simulink model "Copy_of_read_ADC_scribe_PWM_ROB_1ver"  (R2024a)
settings: Solver=ode8  StartTime=0.0  StopTime=400  FixedStep=Ts  RelTol=1e-3  EnableMultiTasking=on
values from neighbouring files (symbols this model uses):
  am = 200    [parameters.m]
  bm = 1    [parameters.m]
  C = 790*10^(-6)    (= 0.00079)    [parameters.m]
  k1 = 8000    [parameters.m]
  k2 = 15    [parameters.m]
  kapam = 1    [parameters.m]
  L = 2000*10^(-6)    (= 0.002)    [parameters.m]
  Qaster = bm    (= 1)    [parameters.m]
  R = 10000    [parameters.m]
  Ts = 0.01    [parameters.m]
  x2d_dot = 0    [parameters.m]
undefined symbols (not defined in the file or in its folder): Down, GPTRIP1SEL, GPTRIP2SEL, TZ1, TZ2, Up
libraries: c2802xlib x5
settings Model: SimulationMode=external  ExtModeTrigDuration=8  Creator=omar_  LastModifiedBy=rodol
settings DataIOCC: LimitDataPoints=on  MaxDataPoints=1000000  SaveFormat=StructureWithTime  InspectSignalLogs=on
settings OptimizationCC: DefaultUnderspecifiedDataType=single  EnhancedBackFolding=on  PassReuseOutputArgsAs=Individual arguments  MaxStackSize=1024  OptimizeBlockOrder=speed  DifferentSizesBufferReuse=on  OptimizationCustomize=off  DenormalBehavior=FlushToZero  EfficientTunableParamExpr=on
settings DebuggingCC: ParameterTunabilityLossMsg=error  UnconnectedInputMsg=warning  UnconnectedOutputMsg=warning  UnconnectedLineMsg=warning
settings HardwareCC: ProdBitPerChar=16  ProdBitPerInt=16  ProdBitPerPointer=32  ProdBitPerSizeT=32  ProdBitPerPtrDiffT=32  ProdLargestAtomicInteger=Integer  ProdLargestAtomicFloat=None  ProdWordSize=16  ProdLongLongMode=on  ProdHWDeviceType=Texas Instruments->C2000
settings ModelReferenceCC: EnableRefExpFcnMdlSchedulingChecks=on
settings SFSimCC: MATLABDynamicMemAlloc=off
settings RTWCC: Description=Embedded Coder  SystemTargetFile=ert.tlc  HardwareBoard=TI Delfino F28379D LaunchPad  TemplateMakefile=ert_default_tmf  Toolchain=Texas Instruments Code Composer Studio (C2000)  GPUComputeCapability=3.5  DLArmComputeVersion=19.05
settings CodeAppCC: ForceParamTrailComments=on  IgnoreCustomStorageClasses=off  OperatorAnnotations=on  SimulinkDataObjDesc=on  SFDataObjDesc=on  InsertBlockDesc=on
settings ERTTargetCC: CodeReplacementLibrary=TI C28x  SupportContinuousTime=on  ExtMode=on  ExtModeTransport=3  ExtModeStaticAllocSize=10000  ExtModeMexArgs='127.0.0.1' 0 17725

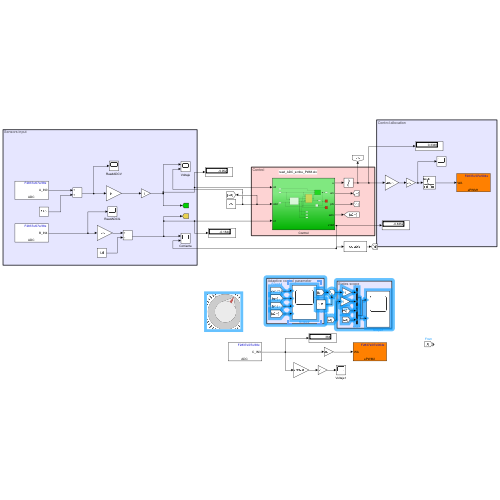
[thumbnail: Simulink's stored preview of the top-level diagram]
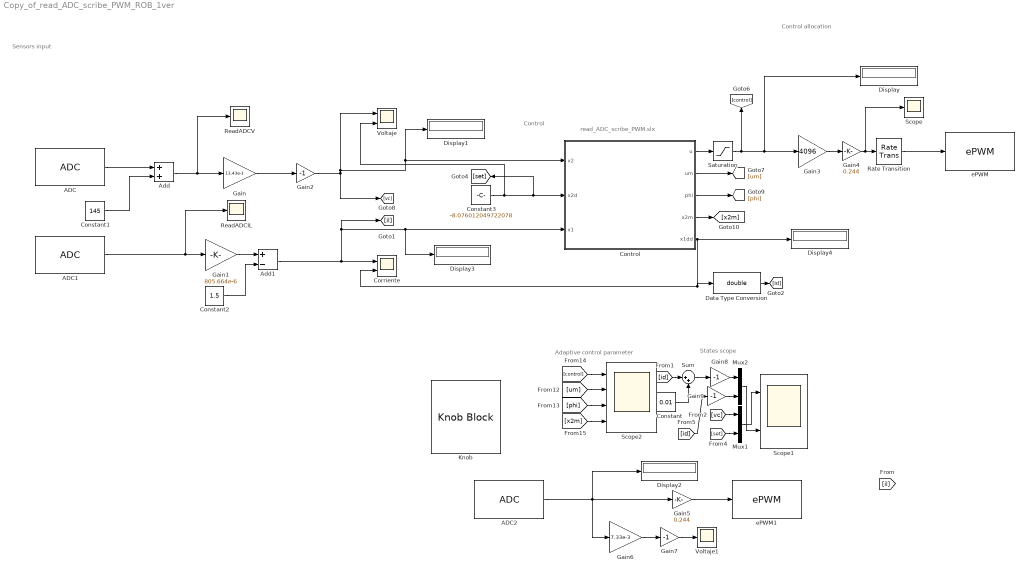
== system Copy_of_read_ADC_scribe_PWM_ROB_1ver ==
  note: Sensors input
  note: Control allocation
  note: read_ADC_scribe_PWM.slx
  note: Control
  note: Adaptive control parameter
  note: States scope
  ADC : c2802xlib/ADC  blkParamProc=C2000_Type4  ADCModule=A  samplingMode=Single sample mode  ADCResolution=12-bit (Single-ended input)  useSOC1=SOC0  useSOC2=SOC0_SOC1  SOCAcquisitionWindow=15  SOCTriggerSource=Software  SOCInterruptTrigger=No ADCINT  Ts=Ts  dType=uint16  postInterrupt=off  interruptSel=ADCINT1  ADCINTContinuous=on  endma=off  chdma=1  conv1=ADCINA0  conv2=ADCINA0 and ADCINB0  conv1_Type4=ADCIN0  conv2_Type4=ADCIN0 and ADCIN1
  ADC1 : c2802xlib/ADC  blkParamProc=C2000_Type4  ADCModule=B  samplingMode=Single sample mode  ADCResolution=12-bit (Single-ended input)  useSOC1=SOC4  useSOC2=SOC0_SOC1  SOCAcquisitionWindow=15  SOCTriggerSource=Software  SOCInterruptTrigger=No ADCINT  Ts=Ts  dType=uint16  postInterrupt=off  interruptSel=ADCINT1  ADCINTContinuous=on  endma=off  chdma=1  conv1=ADCINA0  conv2=ADCINA0 and ADCINB0  conv1_Type4=ADCIN4  conv2_Type4=ADCIN0 and ADCIN1
  ADC2 : c2802xlib/ADC  blkParamProc=C2000_Type4  ADCModule=C  samplingMode=Single sample mode  ADCResolution=12-bit (Single-ended input)  useSOC1=SOC3  useSOC2=SOC0_SOC1  SOCAcquisitionWindow=15  SOCTriggerSource=Software  SOCInterruptTrigger=No ADCINT  Ts=Ts  dType=uint16  postInterrupt=off  interruptSel=ADCINT1  ADCINTContinuous=on  endma=off  chdma=1  conv1=ADCINA0  conv2=ADCINA0 and ADCINB0  conv1_Type4=ADCIN3  conv2_Type4=ADCIN0 and ADCIN1
  Add : Sum
  Add1 : Sum  Inputs=+-
  Constant : Constant  Value=0.01
  Constant1 : Constant  Value=145
  Constant2 : Constant  Value=1.5
  Constant3 : Constant  Value=-8.076012049722078
  Control : Subsystem
  Corriente : Scope  NumInputPorts=2
  Data Type Conversion : DataTypeConversion  OutDataTypeStr=double  SaturateOnIntegerOverflow=off  RndMeth=Floor
  Display{,1..4} (5 alike) : Display
  Gain : Gain  Gain=13.43e-3  ParamDataTypeStr=double
  Gain1 : Gain  Gain=805.664e-6  ParamDataTypeStr=double
  Gain2 : Gain  Gain=-1  ParamDataTypeStr=double
  Gain3 : Gain  Gain=4096
  Gain4 : Gain  Gain=0.244
  Gain5 : Gain  Gain=0.244  OutDataTypeStr=double
  Gain6 : Gain  Gain=7.33e-3  ParamDataTypeStr=double
  Gain7 : Gain  Gain=-1  ParamDataTypeStr=double
  Gain8 : Gain  Gain=-1
  Gain9 : Gain  Gain=-1
  Knob : KnobBlock  ScaleMin=-20  ScaleMax=0
  Mux1 : Mux  Inputs=2
  Mux2 : Mux  Inputs=2
  Rate Transition : RateTransition
  ReadADCIL : Scope
  ReadADCV : Scope
  Saturation : Saturate  UpperLimit=1  LowerLimit=-50
  Scope : Scope
  Scope1 : Scope  NumInputPorts=2
  Scope2 : Scope  NumInputPorts=4
  Sum : Sum  Inputs=|++
  Voltaje : Scope  NumInputPorts=2
  Voltaje1 : Scope
  ePWM : c2802xlib/ePWM  PwmType=C2000_Type4  useModule=ePWM1  ePWMxLINKTBPRD=Not Linked  periodUnits=Clock cycles  timerSource=Specify via dialog  timerPeriod_clk=1000  timerPeriod_sec=0.0001  tbshadow=Counter equals to zero  countingMode=Up-Down  phaseActiveEnable=Disable  phaseDirection=Count down after sync  phaseActive=0  synchronizationEnable=off  dcaevt1Sync=off  dcbevt1Sync=off  synchronizationOption=Disable  dcbevt1SyncOut=off  dcaevt1SyncOut=off  cmpdSyncOut=off  cmpcSyncOut=off  cmpbSyncOut=off  zeroSyncOut=off  swfSyncOut=off  perSynchronizationOption=Counter equals to period (CTR=PRD)  clockPrescale=1  HSclockPrescale=1  enswap=off  ePWMxAStatus=on  ePWMxAactionLogic1=Do nothing  ePWMxAactionLogic2=Do nothing  ePWMxAactionLogic3=Set  ePWMxAactionLogic4=Clear  ePWMxAactionLogic5=Do nothing  ePWMxAactionLogic6=Do nothing  ePWMxACSFenable=off  ePWMxACSFvalue=Forcing disable  ePWMxASFreload=Zero  ePWMxBStatus=on  ePWMxBactionLogic1=Do nothing  ePWMxBactionLogic2=Do nothing  ePWMxBactionLogic3=Do nothing  ePWMxBactionLogic4=Do nothing  ePWMxBactionLogic5=Do nothing  ePWMxBactionLogic6=Do nothing  ePWMxBCSFenable=off  ePWMxBCSFvalue=Forcing disable  ePWMxBSFreload=Zero  ePWNxBOutWay=on  ePWMxLINKCMPA=Not Linked  CMPAUnits=Clock cycles  CMPASource=Input port  CMPAValue_per=50  CMPAValue_clk=5000  enCMPAshadow=Counter equals to zero (CTR=Zero)  ePWMxLINKCMPB=Not Linked  CMPBUnits=Clock cycles  CMPBSource=Specify via dialog  CMPBValue_per=50  CMPBValue_clk=0  enCMPBshadow=Counter equals to zero (CTR=Zero)  ePWMxLINKCMPC=Not Linked  CMPCUnits=Clock cycles  CMPCSource=Specify via dialog  CMPCValue_per=50  CMPCValue_clk=0  enCMPCshadow=Counter equals to zero (CTR=Zero)  ePWMxLINKCMPD=Not Linked  CMPDUnits=Clock cycles  CMPDSource=Specify via dialog  CMPDValue_per=50  CMPDValue_clk=0  enCMPDshadow=Counter equals to zero (CTR=Zero)  enableDBePWMxA=off  enableDBePWMxB=off  enhalfcycle=off  DBpolarity=Active high (AH)  DBedgeDelay=Positive  DBSource_ePWMxA=ePWMxA  DBSource_ePWMxB=ePWMxA  DBPeriodUnits=Clock cycles  DBperiodSource=Specify via dialog  REDperiod=0  FEDperiod=0  REDperiod_sec=0  FEDperiod_sec=0  LoadModeDBRED=Immediate without using shadow  LoadModeDBFED=Immediate without using shadow  adcstartModuleA=on  adcrequestEventA=First event  adcstartEventA=Digital Compare Module A Event 1 start of conversion (DCAEVT1.soc)  adcstartEventA_type2=Counter equals to period (CTR=PRD)  adcstartModuleB=off  adcrequestEventB=First event  adcstartEventB=Counter equals to zero (CTR=Zero)  adcstartEventB_type2=Counter equals to zero (CTR=Zero)  intEn=off  intPrd=First event  intSel=Counter equals to zero (CTR=Zero)  intSel_type2=Counter equals to zero (CTR=Zero)  hrpe=off  enHRPWM=off  HRPWM_LoadMode=Counter equals to period (CTR=PRD)  HRPWM_CTLMode=Duty or Period control mode  HRPWM_EDGMode=Both edge  hrpeb=off  enHRPWMB=off  HRPWM_LoadModeB=Counter equals to zero (CTR=ZERO)  HRPWM_CTLModeB=Duty or Period control mode  HRPWM_EDGModeB=Both edge  enHRDBRED=off  enHRDBFED=off  enSFO=on  enautoconv=on  chopperEnable=off  chopperFrequency=1  chopperFirstwidth=1  chopperDuty=12.5%  tripZonesource=Specify via dialog  tzselOSHT1=off  tzselOSHT2=off  tzselOSHT3=off  tzselOSHT4=off  tzselOSHT5=off  tzselOSHT6=off  tzselOSHDCAEV1=off  tzselOSHDCBEV1=off  tzselCBC1=off  tzselCBC2=off  tzselCBC3=off  tzselCBC4=off  tzselCBC5=off  tzselCBC6=off  tzselCBCDCAEV2=off  tzselCBCDCBEV2=off  enTzOstIntr=off  enTzCbcIntr=off  enTzDCAEVT1Intr=off  enTzDCAEVT2Intr=off  enTzDCBEVT1Intr=off  enTzDCBEVT2Intr=off  tzclrCBCLatch=Counter equals to zero (CTR=Zero)  ePWMxAforced=No action  ePWMxBforced=No action  DCAEVT1forced=No action  DCBEVT1forced=No action  DCAEVT2forced=No action  DCBEVT2forced=No action  dcah=Trip Zone 1 input (TZ1)  dcal=Trip Zone 2 input (TZ2)  dcbh=Trip Zone 1 input (TZ1)  dcbl=Trip Zone 2 input (TZ2)  dcah_type2=GPTRIP1SEL/(TZ1)  dcal_type2=GPTRIP2SEL/(TZ2)  dcbh_type2=GPTRIP1SEL/(TZ1)  dcbl_type2=GPTRIP2SEL/(TZ2)  gendcaevt1=Event disabled  gendcaevt2=Event disabled  gendcbevt1=Event disabled  gendcbevt2=Event disabled  dcaevt1src=DCAEVT1 with sync  dcaevt2src=DCAEVT2 with sync  dcbevt1src=DCBEVT1 with sync  dcbevt2src=DCBEVT2 with sync  pulsesel=Counter equals to zero (CTR=Zero)  blankinv=off  blankoffset=0  blankwidth=0  evsrcsel=Filtered version of DCAEVT1 (DCAEVT1FILT)  encape=off
  ePWM1 : c2802xlib/ePWM  PwmType=C2000_Type4  useModule=ePWM2  ePWMxLINKTBPRD=Not Linked  periodUnits=Clock cycles  timerSource=Specify via dialog  timerPeriod_clk=1000  timerPeriod_sec=0.0001  tbshadow=Counter equals to zero  countingMode=Up-Down  phaseActiveEnable=Disable  phaseDirection=Count down after sync  phaseActive=0  synchronizationEnable=off  dcaevt1Sync=off  dcbevt1Sync=off  synchronizationOption=Disable  dcbevt1SyncOut=off  dcaevt1SyncOut=off  cmpdSyncOut=off  cmpcSyncOut=off  cmpbSyncOut=off  zeroSyncOut=off  swfSyncOut=off  perSynchronizationOption=Counter equals to period (CTR=PRD)  clockPrescale=1  HSclockPrescale=1  enswap=off  ePWMxAStatus=on  ePWMxAactionLogic1=Do nothing  ePWMxAactionLogic2=Do nothing  ePWMxAactionLogic3=Set  ePWMxAactionLogic4=Clear  ePWMxAactionLogic5=Do nothing  ePWMxAactionLogic6=Do nothing  ePWMxACSFenable=off  ePWMxACSFvalue=Forcing disable  ePWMxASFreload=Zero  ePWMxBStatus=on  ePWMxBactionLogic1=Do nothing  ePWMxBactionLogic2=Do nothing  ePWMxBactionLogic3=Do nothing  ePWMxBactionLogic4=Do nothing  ePWMxBactionLogic5=Do nothing  ePWMxBactionLogic6=Do nothing  ePWMxBCSFenable=off  ePWMxBCSFvalue=Forcing disable  ePWMxBSFreload=Zero  ePWNxBOutWay=on  ePWMxLINKCMPA=Not Linked  CMPAUnits=Clock cycles  CMPASource=Input port  CMPAValue_per=50  CMPAValue_clk=5000  enCMPAshadow=Counter equals to zero (CTR=Zero)  ePWMxLINKCMPB=Not Linked  CMPBUnits=Clock cycles  CMPBSource=Specify via dialog  CMPBValue_per=50  CMPBValue_clk=0  enCMPBshadow=Counter equals to zero (CTR=Zero)  ePWMxLINKCMPC=Not Linked  CMPCUnits=Clock cycles  CMPCSource=Specify via dialog  CMPCValue_per=50  CMPCValue_clk=0  enCMPCshadow=Counter equals to zero (CTR=Zero)  ePWMxLINKCMPD=Not Linked  CMPDUnits=Clock cycles  CMPDSource=Specify via dialog  CMPDValue_per=50  CMPDValue_clk=0  enCMPDshadow=Counter equals to zero (CTR=Zero)  enableDBePWMxA=off  enableDBePWMxB=off  enhalfcycle=off  DBpolarity=Active high (AH)  DBedgeDelay=Positive  DBSource_ePWMxA=ePWMxA  DBSource_ePWMxB=ePWMxA  DBPeriodUnits=Clock cycles  DBperiodSource=Specify via dialog  REDperiod=0  FEDperiod=0  REDperiod_sec=0  FEDperiod_sec=0  LoadModeDBRED=Immediate without using shadow  LoadModeDBFED=Immediate without using shadow  adcstartModuleA=on  adcrequestEventA=First event  adcstartEventA=Digital Compare Module A Event 1 start of conversion (DCAEVT1.soc)  adcstartEventA_type2=Counter equals to period (CTR=PRD)  adcstartModuleB=off  adcrequestEventB=First event  adcstartEventB=Counter equals to zero (CTR=Zero)  adcstartEventB_type2=Counter equals to zero (CTR=Zero)  intEn=off  intPrd=First event  intSel=Counter equals to zero (CTR=Zero)  intSel_type2=Counter equals to zero (CTR=Zero)  hrpe=off  enHRPWM=off  HRPWM_LoadMode=Counter equals to period (CTR=PRD)  HRPWM_CTLMode=Duty or Period control mode  HRPWM_EDGMode=Both edge  hrpeb=off  enHRPWMB=off  HRPWM_LoadModeB=Counter equals to zero (CTR=ZERO)  HRPWM_CTLModeB=Duty or Period control mode  HRPWM_EDGModeB=Both edge  enHRDBRED=off  enHRDBFED=off  enSFO=on  enautoconv=on  chopperEnable=off  chopperFrequency=1  chopperFirstwidth=1  chopperDuty=12.5%  tripZonesource=Specify via dialog  tzselOSHT1=off  tzselOSHT2=off  tzselOSHT3=off  tzselOSHT4=off  tzselOSHT5=off  tzselOSHT6=off  tzselOSHDCAEV1=off  tzselOSHDCBEV1=off  tzselCBC1=off  tzselCBC2=off  tzselCBC3=off  tzselCBC4=off  tzselCBC5=off  tzselCBC6=off  tzselCBCDCAEV2=off  tzselCBCDCBEV2=off  enTzOstIntr=off  enTzCbcIntr=off  enTzDCAEVT1Intr=off  enTzDCAEVT2Intr=off  enTzDCBEVT1Intr=off  enTzDCBEVT2Intr=off  tzclrCBCLatch=Counter equals to zero (CTR=Zero)  ePWMxAforced=No action  ePWMxBforced=No action  DCAEVT1forced=No action  DCBEVT1forced=No action  DCAEVT2forced=No action  DCBEVT2forced=No action  dcah=Trip Zone 1 input (TZ1)  dcal=Trip Zone 2 input (TZ2)  dcbh=Trip Zone 1 input (TZ1)  dcbl=Trip Zone 2 input (TZ2)  dcah_type2=GPTRIP1SEL/(TZ1)  dcal_type2=GPTRIP2SEL/(TZ2)  dcbh_type2=GPTRIP1SEL/(TZ1)  dcbl_type2=GPTRIP2SEL/(TZ2)  gendcaevt1=Event disabled  gendcaevt2=Event disabled  gendcbevt1=Event disabled  gendcbevt2=Event disabled  dcaevt1src=DCAEVT1 with sync  dcaevt2src=DCAEVT2 with sync  dcbevt1src=DCBEVT1 with sync  dcbevt2src=DCBEVT2 with sync  pulsesel=Counter equals to zero (CTR=Zero)  blankinv=off  blankoffset=0  blankwidth=0  evsrcsel=Filtered version of DCAEVT1 (DCAEVT1FILT)  encape=off
  wires:
  ADC1/1 -> Gain1/1, ReadADCIL/1
  Gain/1 -> Gain2/1
  Rate Transition/1 -> ePWM/1
  Gain2/1 -> [vc], Display1/1, Control/1(x2), Voltaje/1
  Gain3/1 -> Gain4/1
  Gain4/1 -> Scope/1, Rate Transition/1
  Gain6/1 -> Gain7/1
  Gain5/1 -> ePWM1/1
  Gain7/1 -> Voltaje1/1
  ADC2/1 -> Display2/1, Gain5/1, Gain6/1
  ADC/1 -> Add/1
  Add/1 -> ReadADCV/1, Gain/1
  Constant1/1 -> Add/2
  Gain1/1 -> Add1/1
  Add1/1 -> Display3/1, Control/3(x1), [il], Corriente/1
  Constant2/1 -> Add1/2
  Control/1(u) -> Saturation/1
  Control/3(phi) -> [phi]
  Control/2(um) -> [um]
  Control/4(x2m) -> [x2m]
  Constant3/1 -> Voltaje/2, Control/2(x2d), [set]
  [vc] -> Mux1/1
  [set] -> Mux1/2
  Control/5(x1dd) -> Display4/1, Data Type Conversion/1, Corriente/2
  Data Type Conversion/1 -> [id]
  [control] -> Scope2/1
  [um] -> Scope2/2
  [phi] -> Scope2/3
  [x2m] -> Scope2/4
  Mux2/1 -> Scope1/2
  Mux1/1 -> Scope1/1
  Saturation/1 -> [control], Display/1, Gain3/1
  Gain8/1 -> Mux2/1
  [id] -> Gain9/1
  Gain9/1 -> Mux2/2
  Sum/1 -> Gain8/1
  [id] -> Sum/1
  Constant/1 -> Sum/2

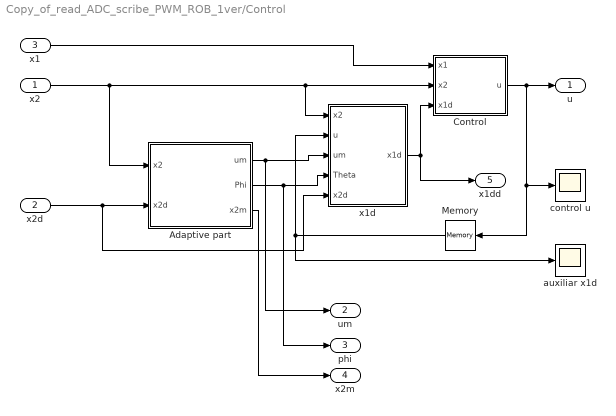
== system Copy_of_read_ADC_scribe_PWM_ROB_1ver/Control ==
  x2 : Inport
  x2d : Inport  Port=2
  x1 : Inport  Port=3
  Adaptive part : Subsystem
  Control : MATLAB Function  TreatAsAtomicUnit=on
  Memory : Memory
  auxiliar x1d : Scope
  control u : Scope
  x1d : MATLAB Function  TreatAsAtomicUnit=on
  u : Outport
  um : Outport  Port=2
  phi : Outport  Port=3
  x2m : Outport  Port=4
  x1dd : Outport  Port=5
  wires:
  x1d/1(x1d) -> x1dd/1, Control/3(x1d)
  Control/1(u) -> control u/1, Memory/1, u/1
  x1/1 -> Control/1(x1)
  x2/1 -> Adaptive part/1(x2), x1d/1(x2), Control/2(x2)
  Memory/1 -> x1d/2(u), auxiliar x1d/1
  Adaptive part/1(um) -> um/1, x1d/3(um)
  Adaptive part/2(Phi) -> phi/1, x1d/4(Theta)
  x2d/1 -> x1d/5(x2d), Adaptive part/2(x2d)
  Adaptive part/3(x2m) -> x2m/1

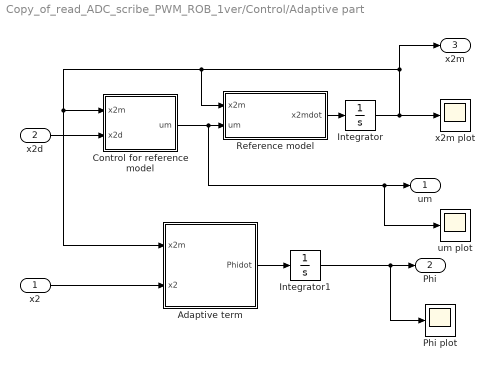
== system Copy_of_read_ADC_scribe_PWM_ROB_1ver/Control/Adaptive part ==
  x2 : Inport
  x2d : Inport  Port=2
  " Control for reference model" : MATLAB Function  TreatAsAtomicUnit=on
  Adaptive term : MATLAB Function  TreatAsAtomicUnit=on
  Integrator : Integrator
  Integrator1 : Integrator
  Phi plot : Scope
  Reference model : MATLAB Function  TreatAsAtomicUnit=on
  um plot : Scope
  x2m plot : Scope
  um : Outport
  Phi : Outport  Port=2
  x2m : Outport  Port=3
  wires:
  Reference model/1(x2mdot) -> Integrator/1
  Integrator/1 -> x2m plot/1, Adaptive term/1(x2m), " Control for reference model"/1(x2m), Reference model/1(x2m), x2m/1
  " Control for reference model"/1(um) -> um plot/1, um/1, Reference model/2(um)
  Adaptive term/1(Phidot) -> Integrator1/1
  Integrator1/1 -> Phi plot/1, Phi/1
  x2/1 -> Adaptive term/2(x2)
  x2d/1 -> " Control for reference model"/2(x2d)

== matlab function Copy_of_read_ADC_scribe_PWM_ROB_1ver/Control/Control ==
  data: x1 input; u output; x2 input; x1d input; E parameter; R parameter; C parameter; L parameter; k1 parameter; k2 parameter
function u = control(x1, x2, x1d, E, R, C, L, k1, k2)

%error
e1 = x1 - x1d;


%control
%u = ( E + k1*L*sign(e1) ) / ( x2 - E) + 1 ;
%u = ( E + k1*L*(e1) ) / ( x2 - E) + 1 ;
u = sigma( L * (k1 * sqrt(abs(e1)) * sign(e1) + E) / (x2 - E) + 1 );

== matlab function Copy_of_read_ADC_scribe_PWM_ROB_1ver/Control/x1d ==
  data: x1d output; x2 input; u input; um input; Theta input; k2 parameter; C parameter; bm parameter; Qaster parameter; x2d input
function x1d = des(x2, u, um, Theta, k2, C, bm, Qaster, x2d)

%error
e2 = x2 - x2d;

%Auxiliar control

%x1d = (( - C*Theta*x2 - C*Qaster*um + k2*C*sign(e2) ) / (1-u))+ 0.001;
%x1d = (( - C*Theta*x2 - C*Qaster*um + k2*C*(e2) ) / (1-u))+ 0.0001;
%x1d = (( - C*Theta*x2 - C*Qaster*um + k2*C*sign(e2) ) / (1-u));
x1d = C * (k2 * sqrt(abs(e2)) * sign(e2) - Theta * x2 - bm * um) / (1 - u);

== matlab function Copy_of_read_ADC_scribe_PWM_ROB_1ver/Control/Adaptive part/Adaptive term ==
  data: x2m input; x2 input; Phidot output; lambda parameter
function Phidot = adaptive(x2m, x2, lambda)

%error:
e2 = x2 - x2m;

%Adaptive Law:
Phidot = - lambda*e2*x2;

== matlab function Copy_of_read_ADC_scribe_PWM_ROB_1ver/Control/Adaptive part/ Control for reference model ==
  data: x2m input; um output; x2d_dot parameter; am parameter; bm parameter; kapam parameter; x2d input
function um = MRC(x2m, x2d_dot, am, bm, kapam, x2d)

um = (1/bm) * ( x2d_dot + am * x2m - kapam * (x2m - x2d) );

== matlab function Copy_of_read_ADC_scribe_PWM_ROB_1ver/Control/Adaptive part/Reference model ==
  data: x2m input; x2mdot output; um input; bm parameter; am parameter
function x2mdot = mrsystem(x2m, um, bm, am)

x2mdot = - am * x2m  +  bm * um ;
